simulink model "zadanie_dodatkowe"  (R2023a)
settings: Solver=VariableStepAuto  StartTime=0.0  StopTime=30  RelTol=1e-3
values from neighbouring files (symbols this model uses):
  K1 = acker(Ar, 1.5*Br, [sb, sb, sb, sb])    [zad_dodatkowe.m]
settings Model: Creator=adams  LastModifiedBy=adams

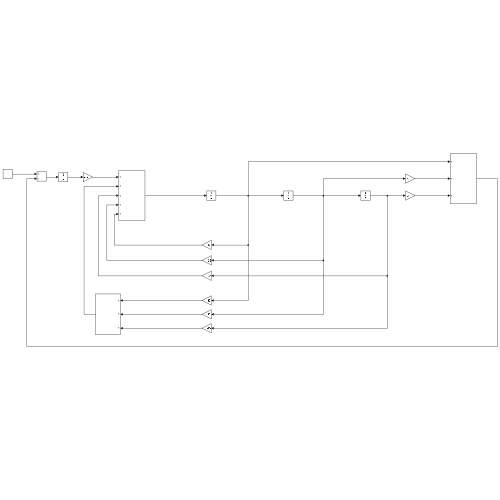
[thumbnail: Simulink's stored preview of the top-level diagram]
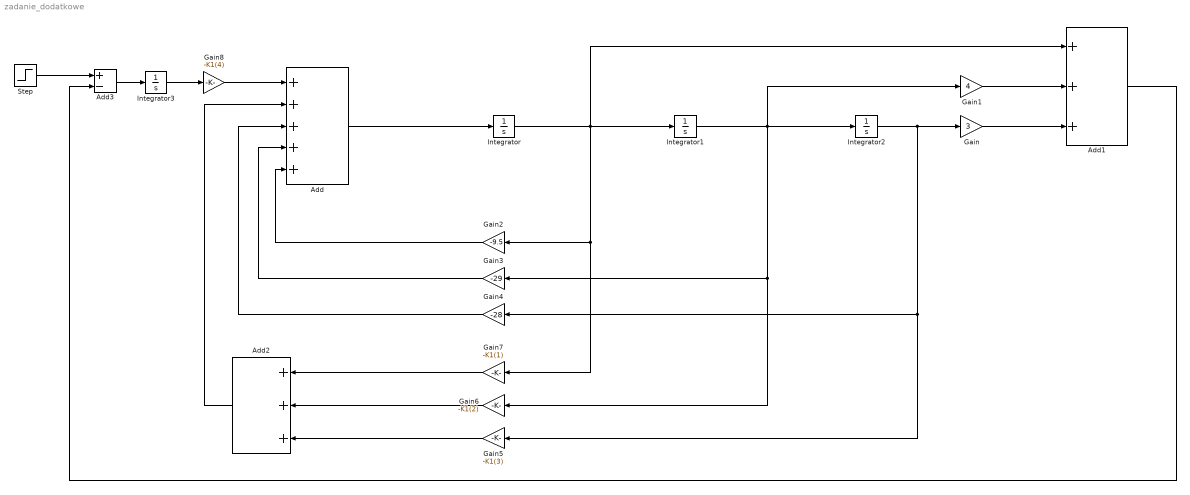
== system zadanie_dodatkowe ==
  Add : Sum  Inputs=+++++
  Add1 : Sum  Inputs=+++
  Add2 : Sum  Inputs=+++
  Add3 : Sum  Inputs=+-
  Gain : Gain  Gain=3
  Gain1 : Gain  Gain=4
  Gain2 : Gain  Gain=-9.5
  Gain3 : Gain  Gain=-29
  Gain4 : Gain  Gain=-28
  Gain5 : Gain  Gain=-K1(3)
  Gain6 : Gain  Gain=-K1(2)
  Gain7 : Gain  Gain=-K1(1)
  Gain8 : Gain  Gain=-K1(4)
  Integrator{,1..3} (4 alike) : Integrator
  Step : Step  SampleTime=0
  wires:
  Gain5/1 -> Add2/3
  Gain6/1 -> Add2/2
  Gain/1 -> Add1/3
  Gain7/1 -> Add2/1
  Integrator/1 -> Gain7/1, Gain2/1, Add1/1, Integrator1/1
  Integrator1/1 -> Integrator2/1, Gain6/1, Gain3/1, Gain1/1
  Add1/1 -> Add3/2
  Gain1/1 -> Add1/2
  Integrator2/1 -> Gain5/1, Gain4/1, Gain/1
  Add/1 -> Integrator/1
  Add3/1 -> Integrator3/1
  Integrator3/1 -> Gain8/1
  Gain2/1 -> Add/5
  Gain3/1 -> Add/4
  Gain4/1 -> Add/3
  Add2/1 -> Add/2
  Gain8/1 -> Add/1
  Step/1 -> Add3/1
